simulink model "eng_mdl_demo_v14"  (Simulink 7.0)
settings: Solver=ode3  StartTime=0.0  StopTime=100  FixedStep=0.001  RelTol=1e-3
PreLoadFcn:
  | eng_mdl_demo_v14_setup
InitFcn:
  | eng_mdl_demo_v14_setup
undefined symbols (not defined in the file or in its folder): notex
libraries: hil14_mdl_lib x1, ni_annotations_lib x1
CloseFcn:
  | eng_mdl_demo_v14_close
settings Model: Creator=Eric Bradley  LastModifiedBy=Eric Bradley
settings OptimizationCC: SimCompilerOptimization=On
settings DebuggingCC: InheritedTsInSrcMsg=none  ParameterPrecisionLossMsg=none
settings RTWCC: SystemTargetFile=NIVeriStand.tlc  TemplateMakefile=NIVeriStand_vc.tmf  Description=NI VeriStand Real-Time Target for Release 2007b or later  ProcessScript=NIVeriStand_make_rtw_hook
settings STFCustomTargetCC: GenFloatMathFcnCalls=ANSI_C  MatFileLogging=on  SystemTargetFile=NIVeriStand.tlc
settings CustomProperty: Value=on
settings EnumStrPairs: String=Default

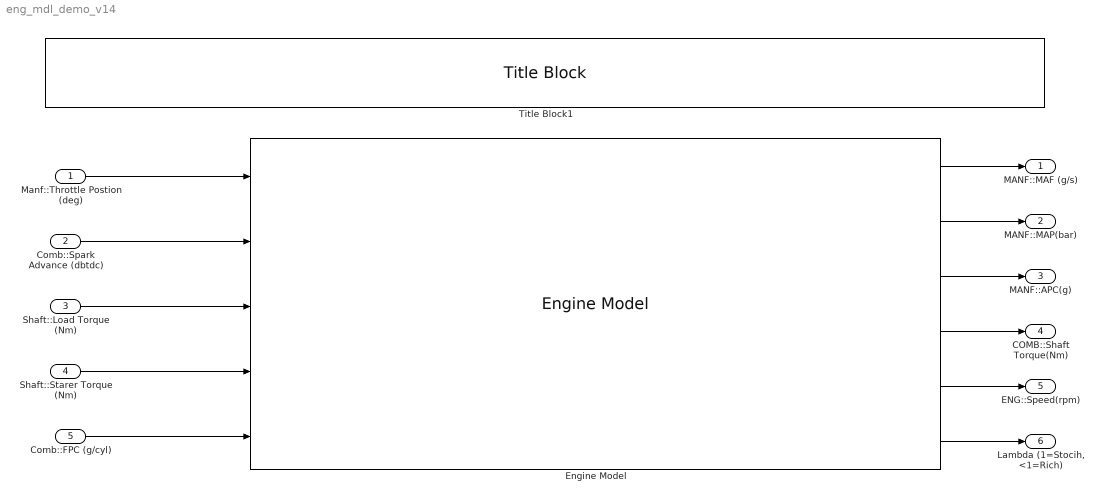
== system eng_mdl_demo_v14 ==
  Manf::Throttle Postion (deg) : Inport  OutDataType=sfix(16)  OutScaling=2^0
  Comb::Spark Advance (dbtdc) : Inport  Port=2  OutDataType=sfix(16)  OutScaling=2^0
  Shaft::Load Torque (Nm) : Inport  Port=3  OutDataType=sfix(16)  OutScaling=2^0
  Shaft::Starer Torque (Nm) : Inport  Port=4  OutDataType=sfix(16)  OutScaling=2^0
  Comb::FPC (g/cyl) : Inport  Port=5  OutDataType=sfix(16)  OutScaling=2^0
  Engine Model : hil14_mdl_lib/Engine Model  SystemSampleTime=-1  iname='engine.jpg'
  Title Block1 : ni_annotations_lib/Title Block  SystemSampleTime=-1  tx_title=notex(get_param(gcs,'Name'))
  MANF::MAF (g/s) : Outport  OutDataType=sfix(16)  OutScaling=2^0
  MANF::MAP(bar) : Outport  Port=2  OutDataType=sfix(16)  OutScaling=2^0
  MANF::APC(g) : Outport  Port=3  OutDataType=sfix(16)  OutScaling=2^0
  COMB::Shaft Torque(Nm) : Outport  Port=4  OutDataType=sfix(16)  OutScaling=2^0
  ENG::Speed(rpm) : Outport  Port=5  OutDataType=sfix(16)  OutScaling=2^0
  "Lambda (1=Stocih, <1=Rich)" : Outport  Port=6  OutDataType=sfix(16)  OutScaling=2^0
  wires:
  Engine Model/5 -> ENG::Speed(rpm)/1
  Engine Model/4 -> COMB::Shaft Torque(Nm)/1
  Engine Model/3 -> MANF::APC(g)/1
  Engine Model/2 -> MANF::MAP(bar)/1
  Engine Model/1 -> MANF::MAF (g/s)/1
  Manf::Throttle Postion (deg)/1 -> Engine Model/1
  Comb::Spark Advance (dbtdc)/1 -> Engine Model/2
  Comb::FPC (g/cyl)/1 -> Engine Model/5
  Shaft::Load Torque (Nm)/1 -> Engine Model/3
  Shaft::Starer Torque (Nm)/1 -> Engine Model/4
  Engine Model/6 -> "Lambda (1=Stocih, <1=Rich)"/1
